simulink model "PB3_DCS_810698349"  (R2021b)
settings: Solver=VariableStepAuto  StartTime=0.0  StopTime=10  FixedStep=0.001*Ts  RelTol=1e-3
undefined symbols (not defined in the file or in its folder): Dd, e_ss, g, K, L, M, R, Ts, y0, y00
settings Model: Creator=SinaK  LastModifiedBy=SinaK

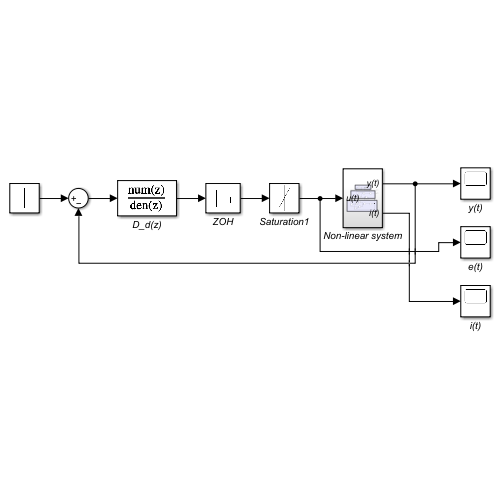
[thumbnail: Simulink's stored preview of the top-level diagram]
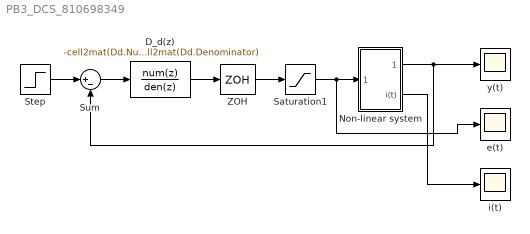
== system PB3_DCS_810698349 ==
  D_d(z) : DiscreteTransferFcn  Numerator=-cell2mat(Dd.Numerator)  Denominator=cell2mat(Dd.Denominator)  SampleTime=Ts
  Non-linear system : Subsystem
  Saturation1 : Saturate  UpperLimit=12  LowerLimit=0
  Step : Step  Time=0  After=y0/e_ss  SampleTime=Ts
  Sum : Sum  Inputs=|+-
  ZOH : ZeroOrderHold  SampleTime=Ts
  e(t) : Scope
  i(t) : Scope
  y(t) : Scope
  wires:
  Step/1 -> Sum/1
  Sum/1 -> D_d(z)/1
  Non-linear system/1(y(t)) -> Sum/2, y(t)/1
  Non-linear system/2(i(t)) -> i(t)/1
  D_d(z)/1 -> ZOH/1
  ZOH/1 -> Saturation1/1
  Saturation1/1 -> e(t)/1, Non-linear system/1(u(t))

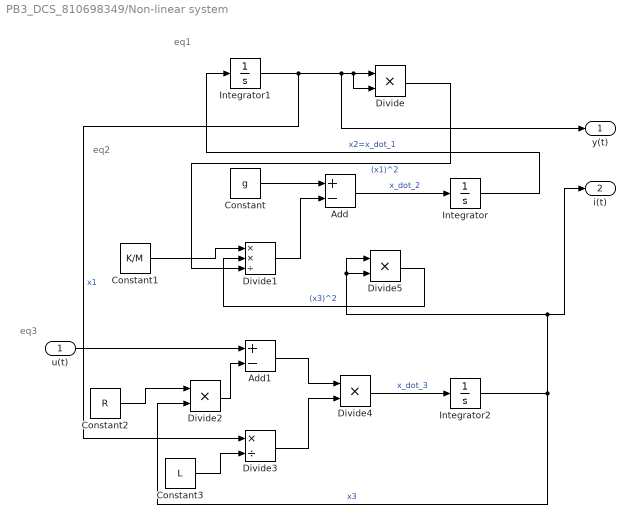
== system PB3_DCS_810698349/Non-linear system ==
  note: eq1
  note: eq2
  note: eq3
  u(t) : Inport
  Add : Sum  Inputs=+-
  Add1 : Sum  Inputs=+-
  Constant : Constant  Value=g  SampleTime=Ts
  Constant1 : Constant  Value=K/M  SampleTime=Ts
  Constant2 : Constant  Value=R  SampleTime=Ts
  Constant3 : Constant  Value=L  SampleTime=Ts
  Divide{,2,4..5} (4 alike) : Product  Inputs=**
  Divide1 : Product  Inputs=**/
  Divide3 : Product  Inputs=*/
  Integrator : Integrator
  Integrator1 : Integrator  InitialCondition=y00
  Integrator2 : Integrator
  y(t) : Outport
  i(t) : Outport  Port=2
  wires:
  Add/1 -> Integrator/1  "x_dot_2"
  Divide/1 -> Divide1/3  "(x1)^2"
  Integrator/1 -> Integrator1/1  "x2=x_dot_1"
  Integrator2/1 -> Divide5/1, Divide5/2, i(t)/1, Divide2/2  "x3"
  Divide1/1 -> Add/2
  Add1/1 -> Divide4/1
  Constant3/1 -> Divide3/2
  Constant2/1 -> Divide2/1
  Divide5/1 -> Divide1/2  "(x3)^2"
  Integrator1/1 -> Divide3/1, y(t)/1, Divide/2, Divide/1  "x1"
  Divide4/1 -> Integrator2/1  "x_dot_3"
  Constant1/1 -> Divide1/1
  Constant/1 -> Add/1
  Divide3/1 -> Divide4/2
  Divide2/1 -> Add1/2
  u(t)/1 -> Add1/1
